simulink model "vj1sim"  (R2020b)
settings: Solver=VariableStepAuto  StartTime=0.0  StopTime=25  RelTol=1e-6
settings Model: Creator=Korisnik  LastModifiedBy=Korisnik

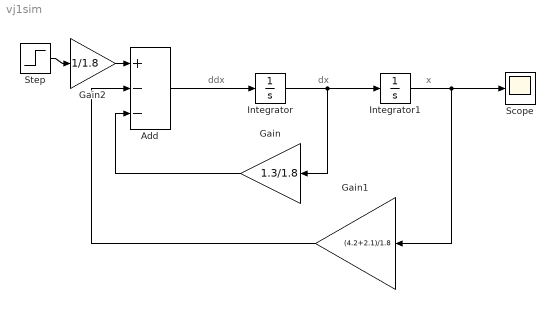
== system vj1sim ==
  note: dx
  note: ddx
  note: x
  Add : Sum  Inputs=+--
  Gain : Gain  Gain=1.3/1.8
  Gain1 : Gain  Gain=(4.2+2.1)/1.8
  Gain2 : Gain  Gain=1/1.8
  Integrator : Integrator
  Integrator1 : Integrator
  Scope : Scope
  Step : Step  Time=0  After=2  SampleTime=0
  wires:
  Integrator/1 -> Gain/1, Integrator1/1
  Integrator1/1 -> Gain1/1, Scope/1
  Add/1 -> Integrator/1
  Gain/1 -> Add/3
  Gain1/1 -> Add/2
  Step/1 -> Gain2/1
  Gain2/1 -> Add/1
